simulink model "deneme"  (R2021a)
settings: Solver=FixedStepDiscrete  StartTime=0.0  StopTime=2  RelTol=1e-3  EnableMultiTasking=on
InitFcn:
  | pull_data ;
model workspace (MAT data in the model file):
  encoderResolution = 2000
  hallOffset = '0.5'
  indexOffset = 850
  polePairs = '4'
values from neighbouring files (symbols this model uses):
  bldc = mcb_bldc_param    [pull_data.m]
  dataType = 'single'    [pull_data.m]
  inverter = mcb_updateInverterParameters(bldc,inverter,target)    [pull_data.m]
  PI_params = mcb.internal.SetControllerParameters(bldc,inverter,PU_System,T_pwm,2*Ts,Ts_speed)    [pull_data.m]
  PU_System = mcb_SetPUSystem(bldc,inverter)    [pull_data.m]
  PWM_frequency = 20e3    (= 20000)    [pull_data.m]
  target = mcb_SetProcessorDetails('F28379D',PWM_frequency)    [pull_data.m]
  Ts = T_pwm    (= 5e-05)    [pull_data.m]
  Ts_motor = T_pwm/2    (= 2.5e-05)    [pull_data.m]
  Ts_motor_simscape = T_pwm/100    (= 5e-07)    [pull_data.m]
  Ts_simulink = T_pwm/2    (= 2.5e-05)    [pull_data.m]
  Ts_speed = 10*Ts    (= 0.0005)    [pull_data.m]
undefined symbols (not defined in the file or in its folder): Down, GPTRIP1SEL, GPTRIP2SEL, TZ1, TZ2, Up
libraries: nesl_utility x15, simulink x14, fl_lib x10, c2802xlib x9, mcbcontrolslib x8, c280xlib x6, mcbpositiondecoderlib x5, c2837xDlib x5, ee_lib x5, c2000lib x1, svdutilitieslib x1
(part 3 of 3)

== system deneme/Current Control/Input Scaling/Convert ADC value to PU/Data_Type/Data_Type_Float ==
  In1 : Inport
  Get ADC Voltage : Gain  Gain=target.ADC_Vref /target.ADC_MaxCount  OutDataTypeStr=dataType  RndMeth=Simplest
  Get Currents : Gain  Gain=1/inverter.ISenseVoltPerAmp  RndMeth=Simplest  OutDataTypeStr=Inherit: Same as input
  PU_Conversion : Gain  Gain=1/PU_System.I_base  RndMeth=Simplest  OutDataTypeStr=Inherit: Same as input
  Iab_meas_PU : Outport
  wires:
  Get ADC Voltage/1 -> Get Currents/1
  Get Currents/1 -> PU_Conversion/1
  In1/1 -> Get ADC Voltage/1
  PU_Conversion/1 -> Iab_meas_PU/1

== system deneme/Current Control/Input Scaling/Hall Feedback/Speed Counter/Enabled Subsystem ==
  In1 : Inport
  Hall_State : Inport  Port=2
  Enable : EnablePort
  Constant4 : Constant  OutDataTypeStr=uint32  SampleTime=-1
  Sum : Sum  Inputs=|++  AccumDataTypeStr=uint32  OutDataTypeStr=uint32  RndMeth=Simplest
  Unit Delay1 : UnitDelay  InitialCondition=1  SampleTime=-1  HasFrameUpgradeWarning=on
  Speed_Count : Outport
  PrevHallState : Outport  Port=2
  wires:
  Sum/1 -> Speed_Count/1
  Constant4/1 -> Sum/2
  In1/1 -> Sum/1
  Hall_State/1 -> Unit Delay1/1
  Unit Delay1/1 -> PrevHallState/1

== system deneme/Current Control/Input Scaling/QEP Feedback/ Calculate Position and Speed/IndexFinder ==
  In1 : Inport
  Enable : EnablePort
  AND : Logic  AllPortsSameDT=off  OutDataTypeStr=boolean
  Compare To Constant : simulink/Logic and Bit Operations/Compare To Constant  relop===  const=0  OutDataTypeStr=boolean
  Compare To Constant1 : simulink/Logic and Bit Operations/Compare To Constant  relop=>  const=0  OutDataTypeStr=boolean
  Delay3 : Delay  DelayLength=1
  Out1 : Outport
  wires:
  In1/1 -> Delay3/1, Compare To Constant1/1
  Compare To Constant1/1 -> AND/2
  Compare To Constant/1 -> AND/1
  Delay3/1 -> Compare To Constant/1
  AND/1 -> Out1/1

== system deneme/Hardware Init/Code Generation/Calculate ADC Offset /For Iterator Subsystem/If Action Subsystem ==
  In1 : Inport
  In2 : Inport  Port=2
  In3 : Inport  Port=3
  Action Port : ActionPort  ActionPortLabel=if(u1 > 8)
  Memory : Memory  InheritSampleTime=on
  Memory1 : Memory  InheritSampleTime=on
  Memory2 : Memory  InheritSampleTime=on
  Sum : Sum
  Sum1 : Sum
  Sum2 : Sum
  Out1 : Outport
  Out2 : Outport  Port=2
  Out3 : Outport  Port=3
  wires:
  In1/1 -> Sum/1
  Sum/1 -> Out1/1, Memory/1
  In2/1 -> Sum1/1
  Memory/1 -> Sum/2
  Sum1/1 -> Out2/1, Memory1/1
  Memory1/1 -> Sum1/2
  Memory2/1 -> Sum2/2
  Sum2/1 -> Out3/1, Memory2/1
  In3/1 -> Sum2/1

== system deneme/Inverter and Motor - Plant Model/Simulation/EE_PWM/Subsystem1/Sensing w a ==
  Hall sensor : Subsystem
  MRRef : fl_lib/Mechanical/Rotational Elements/Mechanical Rotational Reference
  Motion Sensor : fl_lib/Mechanical/Mechanical Sensors/Ideal Rotational Motion Sensor  wrap_angle=simscape.enum.onoff.off  offset=0 deg
  PS-Simulink Converter1 : nesl_utility/PS-Simulink Converter  PhysicalDomain=network_engine_domain  SubClassName=ps_output  LeftPortType=input  RightPortType=output  PseudoPeriodic=off  Frequencies=[]  Unit=rpm  AffineConversion=off
      settings: SourceProductBaseCode=PW,SS
  PS-Simulink Converter2 : nesl_utility/PS-Simulink Converter  PhysicalDomain=network_engine_domain  SubClassName=ps_output  LeftPortType=input  RightPortType=output  PseudoPeriodic=off  Frequencies=[]  Unit=rad  AffineConversion=off
      settings: SourceProductBaseCode=PW,SS
  Terminator : Terminator
  R : PMIOPort  Side=Left
  tag scope: HallSim=global
  wires:
  PS-Simulink Converter1/1 -> Terminator/1
  PS-Simulink Converter2/1 -> Hall sensor/1(theta)
  Hall sensor/1(Hall) -> [HallSim]
  connections:
  R/RConn1 -- Motion Sensor/LConn1
  Motion Sensor/RConn2 -- PS-Simulink Converter1/LConn1
  MRRef/LConn1 -- Motion Sensor/RConn1
  Motion Sensor/RConn3 -- PS-Simulink Converter2/LConn1

== system deneme/Inverter and Motor - Plant Model/Simulation/Sensor_Measurements/Halls/Hall Signals HW ==
  HallState : Inport
  Bitwise AND1 : simulink/Logic and Bit Operations/Bitwise Operator  logicop=AND  UseBitMask=on  BitMask=bin2dec('00000010')  BitMaskRealWorld=Stored Integer
  Bitwise AND2 : simulink/Logic and Bit Operations/Bitwise Operator  logicop=AND  UseBitMask=on  BitMask=bin2dec('00000100')  BitMaskRealWorld=Stored Integer
  Bitwise AND3 : simulink/Logic and Bit Operations/Bitwise Operator  logicop=AND  UseBitMask=on  BitMask=bin2dec('00000001')  BitMaskRealWorld=Stored Integer
  Data Type Conversion : DataTypeConversion  OutDataTypeStr=boolean
  Data Type Conversion1 : DataTypeConversion  OutDataTypeStr=boolean
  Data Type Conversion2 : DataTypeConversion  OutDataTypeStr=boolean
  Mux : Mux  Inputs=3
  Hall Signals : Outport
  wires:
  Mux/1 -> Hall Signals/1
  HallState/1 -> Bitwise AND3/1, Bitwise AND2/1, Bitwise AND1/1
  Data Type Conversion1/1 -> Mux/2
  Bitwise AND1/1 -> Data Type Conversion1/1
  Bitwise AND3/1 -> Data Type Conversion/1
  Bitwise AND2/1 -> Data Type Conversion2/1
  Data Type Conversion/1 -> Mux/3
  Data Type Conversion2/1 -> Mux/1

== system deneme/Inverter and Motor - Plant Model/Simulation/Sensor_Measurements/Halls/Hall State Plant to HW ==
  HallStatePlant : Inport
  Data Type Conversion : DataTypeConversion  OutDataTypeStr=uint8
  If Action Subsystem : Subsystem  TreatAsAtomicUnit=on
  If Action Subsystem1 : Subsystem  TreatAsAtomicUnit=on
  If Action Subsystem2 : Subsystem  TreatAsAtomicUnit=on
  If Action Subsystem3 : Subsystem  TreatAsAtomicUnit=on
  If Action Subsystem4 : Subsystem  TreatAsAtomicUnit=on
  If Action Subsystem5 : Subsystem  TreatAsAtomicUnit=on
  Merge : Merge  Inputs=6
  Switch Case : SwitchCase  CaseConditions={1,5,4,6,2,3}  ShowDefaultCase=off
  HallstateHw : Outport
  wires:
  Merge/1 -> Data Type Conversion/1
  HallStatePlant/1 -> Switch Case/1
  If Action Subsystem3/1(Out1) -> Merge/4
  Switch Case/4 -> If Action Subsystem3/Action
  If Action Subsystem5/1(Out1) -> Merge/6
  Switch Case/1 -> If Action Subsystem/Action
  Switch Case/6 -> If Action Subsystem5/Action
  Switch Case/3 -> If Action Subsystem2/Action
  If Action Subsystem/1(Out1) -> Merge/1
  If Action Subsystem4/1(Out1) -> Merge/5
  Switch Case/5 -> If Action Subsystem4/Action
  If Action Subsystem2/1(Out1) -> Merge/3
  If Action Subsystem1/1(Out1) -> Merge/2
  Switch Case/2 -> If Action Subsystem1/Action
  Data Type Conversion/1 -> HallstateHw/1

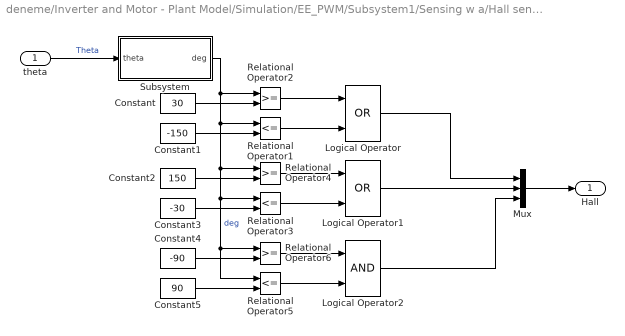
== system deneme/Inverter and Motor - Plant Model/Simulation/EE_PWM/Subsystem1/Sensing w a/Hall sensor ==
  theta : Inport
  Constant : Constant  Value=30
  Constant1 : Constant  Value=-150
  Constant2 : Constant  Value=150
  Constant3 : Constant  Value=-30
  Constant4 : Constant  Value=-90
  Constant5 : Constant  Value=90
  Logical Operator : Logic  Operator=OR  AllPortsSameDT=off  OutDataTypeStr=boolean
  Logical Operator1 : Logic  Operator=OR  AllPortsSameDT=off  OutDataTypeStr=boolean
  Logical Operator2 : Logic  AllPortsSameDT=off  OutDataTypeStr=boolean
  Mux : Mux  Inputs=3
  Relational Operator1 : RelationalOperator  Operator=<=  RndMeth=Nearest  InputSameDT=on
  Relational Operator2 : RelationalOperator  RndMeth=Nearest  InputSameDT=on
  Relational Operator3 : RelationalOperator  Operator=<=  RndMeth=Nearest  InputSameDT=on
  Relational Operator4 : RelationalOperator  RndMeth=Nearest  InputSameDT=on
  Relational Operator5 : RelationalOperator  Operator=<=  RndMeth=Nearest  InputSameDT=on
  Relational Operator6 : RelationalOperator  RndMeth=Nearest  InputSameDT=on
  Subsystem : Subsystem
  Hall : Outport  VectorParamsAs1DForOutWhenUnconnected=off
  wires:
  theta/1 -> Subsystem/1(theta)  "Theta"
  Constant2/1 -> Relational Operator4/2
  Constant1/1 -> Relational Operator1/2
  Relational Operator4/1 -> Logical Operator1/1
  Constant/1 -> Relational Operator2/2
  Subsystem/1(deg) -> Relational Operator2/1, Relational Operator1/1, Relational Operator6/1, Relational Operator5/1, Relational Operator3/1, Relational Operator4/1  "deg"
  Relational Operator1/1 -> Logical Operator/2
  Relational Operator2/1 -> Logical Operator/1
  Mux/1 -> Hall/1
  Relational Operator3/1 -> Logical Operator1/2
  Constant5/1 -> Relational Operator5/2
  Constant4/1 -> Relational Operator6/2
  Relational Operator6/1 -> Logical Operator2/1
  Relational Operator5/1 -> Logical Operator2/2
  Logical Operator/1 -> Mux/1
  Logical Operator1/1 -> Mux/2
  Logical Operator2/1 -> Mux/3
  Constant3/1 -> Relational Operator3/2

== system deneme/Inverter and Motor - Plant Model/Simulation/Sensor_Measurements/Halls/Hall State Plant to HW/If Action Subsystem ==
  Action Port : ActionPort  ActionPortLabel=case [ 1 ]:
  Constant : Constant  Value=bldc.HallSequence(1)  OutDataTypeStr=uint16
  Out1 : Outport
  wires:
  Constant/1 -> Out1/1

== system deneme/Inverter and Motor - Plant Model/Simulation/Sensor_Measurements/Halls/Hall State Plant to HW/If Action Subsystem1 ==
  Action Port : ActionPort  ActionPortLabel=case [ 5 ]:
  Constant : Constant  Value=bldc.HallSequence(2)  OutDataTypeStr=uint16
  Out1 : Outport
  wires:
  Constant/1 -> Out1/1

== system deneme/Inverter and Motor - Plant Model/Simulation/Sensor_Measurements/Halls/Hall State Plant to HW/If Action Subsystem2 ==
  Action Port : ActionPort  ActionPortLabel=case [ 4 ]:
  Constant : Constant  Value=bldc.HallSequence(3)  OutDataTypeStr=uint16
  Out1 : Outport
  wires:
  Constant/1 -> Out1/1

== system deneme/Inverter and Motor - Plant Model/Simulation/Sensor_Measurements/Halls/Hall State Plant to HW/If Action Subsystem3 ==
  Action Port : ActionPort  ActionPortLabel=case [ 6 ]:
  Constant : Constant  Value=bldc.HallSequence(4)  OutDataTypeStr=uint16
  Out1 : Outport
  wires:
  Constant/1 -> Out1/1

== system deneme/Inverter and Motor - Plant Model/Simulation/Sensor_Measurements/Halls/Hall State Plant to HW/If Action Subsystem4 ==
  Action Port : ActionPort  ActionPortLabel=case [ 2 ]:
  Constant : Constant  Value=bldc.HallSequence(5)  OutDataTypeStr=uint16
  Out1 : Outport
  wires:
  Constant/1 -> Out1/1

== system deneme/Inverter and Motor - Plant Model/Simulation/Sensor_Measurements/Halls/Hall State Plant to HW/If Action Subsystem5 ==
  Action Port : ActionPort  ActionPortLabel=case [ 3 ]:
  Constant : Constant  Value=bldc.HallSequence(6)  OutDataTypeStr=uint16
  Out1 : Outport
  wires:
  Constant/1 -> Out1/1

== system deneme/Inverter and Motor - Plant Model/Simulation/EE_PWM/Subsystem1/Sensing w a/Hall sensor/Subsystem ==
  theta : Inport
  Trigonometric Function : Trigonometry  Operator=sincos
  Trigonometric Function2 : Trigonometry  Operator=atan2
  mech->elec : Gain  Gain=bldc.p
  rad->deg : Gain  Gain=180/pi  SaturateOnIntegerOverflow=on  OutDataTypeStr=Inherit: Same as input  ParamDataTypeStr=Inherit: Same as input
  deg : Outport  VectorParamsAs1DForOutWhenUnconnected=off
  wires:
  mech->elec/1 -> Trigonometric Function/1
  Trigonometric Function/2 -> Trigonometric Function2/2
  rad->deg/1 -> deg/1
  theta/1 -> mech->elec/1
  Trigonometric Function/1 -> Trigonometric Function2/1
  Trigonometric Function2/1 -> rad->deg/1
